simulink model "pid_control_V1"  (R2025b)
settings: Solver=FixedStepAuto  StartTime=0.0  StopTime=tsim  FixedStep=0.01  RelTol=1e-3
values from neighbouring files (symbols this model uses):
  Cp = 0.57    [Model.m]    (also in main_V1.m = 0.248)
  h_sp = 1.0    (= 1)    [main_V1.m]
  Kd_h = 5e-5    (= 5e-05)    [main_V1.m]
  Kd_pitch = 0.5    [main_V1.m]
  Ki_h = 1e-6    (= 1e-06)    [main_V1.m]
  Ki_pitch = 0.005    [main_V1.m]
  Kp_h = 1e-5    (= 1e-05)    [main_V1.m]
  Kp_pitch = 1.0    (= 1)    [main_V1.m]
  theta_sp = 2.5 * (pi/180)    (= 0.0436332312999)    [main_V1.m]
  Tp = 0.125*10^(-3)    (= 0.000125)    [Model.m]    (also in main_V1.m)
  u_nom = zeros(5,1)    [main_V1.m]
  x0 = x_nom    [main_V1.m]
undefined symbols (not defined in the file or in its folder): F, Light, MIL, state
libraries: aerolibactuator x5, ros2lib x2, slpidlib x2, robotcorelib x1, aerolibwind2 x1
settings Model: Creator=sofij  LastModifiedBy=facyu
settings SolverCC: AlgebraicLoopSolver=TrustRegion
settings OptimizationCC: DefaultParameterBehavior=Inlined  EnhancedBackFolding=on  PassReuseOutputArgsAs=Individual arguments  ZeroExternalMemoryAtStartup=off  ZeroInternalMemoryAtStartup=off  MaxStackSize=64  OptimizeBlockOrder=speed  DifferentSizesBufferReuse=on  OptimizationCustomize=off  EfficientTunableParamExpr=on
settings DebuggingCC: ParameterTunabilityLossMsg=error  UnconnectedInputMsg=warning  UnconnectedOutputMsg=warning  UnconnectedLineMsg=warning  SFUnexpectedBacktrackingDiag=warning  SFNoUnconditionalDefaultTransitionDiag=warning
settings HardwareCC: ProdBitPerLong=64.0  ProdHWDeviceType=Intel->x86-64 (Linux 64)  UseEmbeddedCoderFeatures=off
settings ModelReferenceCC: EnableRefExpFcnMdlSchedulingChecks=on
settings SFSimCC: MATLABDynamicMemAlloc=off
settings RTWCC: SystemTargetFile=ert.tlc  HardwareBoard=Robot Operating System 2 (ROS 2)  TLCOptions="-aInlineSetEventsForThisBaseRateFcn=TLC_FALSE -aSuppressMultiTaskScheduler=TLC_FALSE  -aRateBasedStepFcn=0"  TemplateMakefile=ert_default_tmf  GenerateReport=on  Toolchain=Colcon Tools  BuildConfiguration=Debug  LaunchReport=on  TargetLang=C++  GPUComputeCapability=3.5  DLArmComputeVersion=19.05  Description=Embedded Coder
settings CodeAppCC: ForceParamTrailComments=on  IgnoreCustomStorageClasses=off  OperatorAnnotations=on  SimulinkDataObjDesc=on  SFDataObjDesc=on  InsertBlockDesc=on  EnableCustomComments=on
settings ERTTargetCC: ExtModeTransport=2.0  ExtModeStaticAlloc=on  ExtModeAutomaticAllocSize=off  ExtModeMexFile=ext_xcp  ExtModeIntrfLevel=Level2 - Open  RootIOFormat=Structure reference  CodeInterfacePackaging=C++ class  SupportNonInlinedSFcns=on

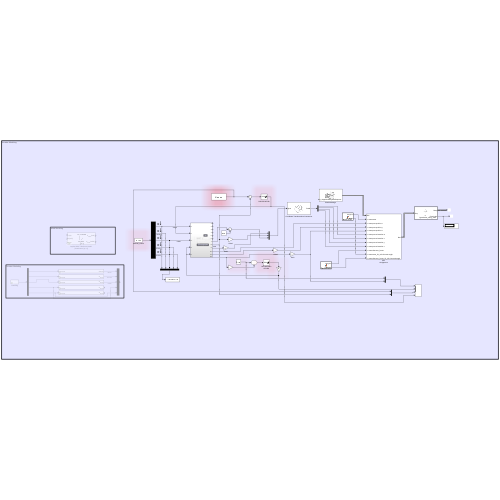
[thumbnail: Simulink's stored preview of the top-level diagram]
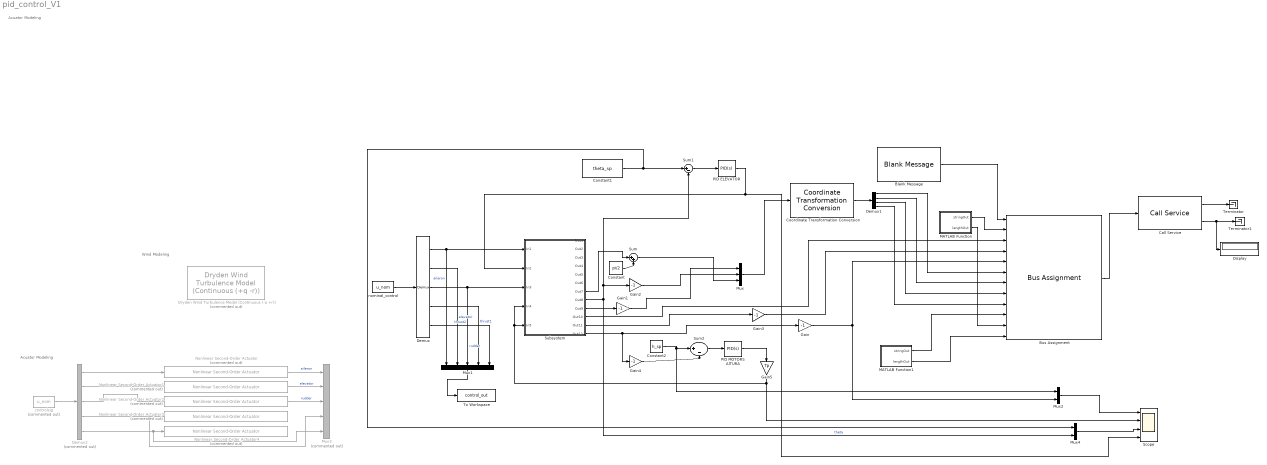
== system pid_control_V1 ==
  note: Wind Modeling
  note: Acuator Modeling
  note: Acuator Modeling
  Blank Message : ros2lib/Blank Message  messageClass=Service Request  entityType=gazebo_msgs/SetEntityState  messageType=gazebo_msgs/SetEntityStateRequest  SampleTime=0.01
  Bus Assignment : BusAssignment  AssignedSignals=state.name,state.pose.position.x,state.pose.position.y,state.pose.position.z,state.pose.orientation.w,state.pose.orientation.z,state.pose.orientation.y,state.pose.orientation.x,state.reference_frame,state.name_SL_Info.CurrentLength,state.reference_frame_SL_Info.CurrentLength
  Call Service : ros2lib/Call Service  topicSource=Specify your own  service=/gazebo/set_entity_state  serviceType=gazebo_msgs/SetEntityState  connectionTimeout=5  ShowErrorCodeOutput=on  legacyBusStruct=off  QOSHistory=Keep last  QOSDepth=1  QOSReliability=Reliable  QOSDurability=Volatile  QOSDeadline=Inf  QOSLifespan=Inf  QOSLiveliness=Automatic  QOSLeaseDuration=Inf  QOSAvoidROSNamespaceConventions=off
  Constant : Constant  Value=pi/2
  Constant1 : Constant  Value=theta_sp
  Constant2 : Constant  Value=h_sp
  Coordinate Transformation Conversion : robotcorelib/Coordinate Transformation Conversion  InputRepresentation=Euler Angles  InputEulerSequence=ZYX  ShowTrVecInputPort=on  OutputRepresentation=Quaternion  OutputEulerSequence=ZYX  ShowTrVecOutputPort=on  SimulateUsing=Interpreted execution
      settings: LibrarySourceBlock=roslib/Utilities/Coordinate Transformation Conversion
  Demux : Demux  Outputs=5
  Demux1 : Demux
  Demux2 : Demux  Commented=on  Outputs=5
  Display : Display
  Dryden Wind Turbulence Model (Continuous (-q +r)) : aerolibwind2/Dryden Wind Turbulence Model  (Continuous (+q -r))  Commented=on  units=Metric (MKS)  spec=MIL-F-8785C  model=Continuous Dryden (-q +r)  W20=15  Wdeg=0  TurbProb=10^-2 - Light  L_high=533.4  Wingspan=10  ts=0.1  Seed=[23341 23342 23343 23344]  T_on=on
  Gain{,1..4} (5 alike) : Gain  Gain=-1
  Gain5 : Gain  Gain=Tp
  MATLAB Function : MATLAB Function  TreatAsAtomicUnit=on
  MATLAB Function1 : MATLAB Function  TreatAsAtomicUnit=on
  Mux : Mux  Inputs=3
  Mux1 : Mux  Inputs=5
  Mux2 : Mux  Inputs=2
  Mux3 : Mux  Commented=on  Inputs=5
  Mux4 : Mux  Inputs=2
  Nonlinear Second-Order Actuator : aerolibactuator/Nonlinear Second-Order Actuator  Commented=on  wn_fin=1  z_fin=0.3  fin_max=15*pi/180  fin_min=-20*pi/180  fin_maxrate=500*pi/180  fin_act_0=0  fin_act_vel=0
  Nonlinear Second-Order Actuator1 : aerolibactuator/Nonlinear Second-Order Actuator  Commented=on  wn_fin=1  z_fin=0.3  fin_max=20*pi/180  fin_min=-20*pi/180  fin_maxrate=500*pi/180  fin_act_0=0  fin_act_vel=0
  Nonlinear Second-Order Actuator2 : aerolibactuator/Nonlinear Second-Order Actuator  Commented=on  wn_fin=1  z_fin=0.3  fin_max=15*pi/180  fin_min=-15*pi/180  fin_maxrate=500*pi/180  fin_act_0=0  fin_act_vel=0
  Nonlinear Second-Order Actuator3 : aerolibactuator/Nonlinear Second-Order Actuator  Commented=on  wn_fin=1  z_fin=0.3  fin_max=100  fin_min=0  fin_maxrate=500*pi/180  fin_act_0=0  fin_act_vel=0
  Nonlinear Second-Order Actuator4 : aerolibactuator/Nonlinear Second-Order Actuator  Commented=on  wn_fin=1  z_fin=0.3  fin_max=100  fin_min=0  fin_maxrate=500*pi/180  fin_act_0=0  fin_act_vel=0
  PID ELEVATOR : slpidlib/PID Controller  Controller=PID  Form=Parallel  TimeDomain=Continuous-time  UseExternalTs=off  SampleTime=-1  IntegratorMethod=Forward Euler  FilterMethod=Forward Euler  ControllerParametersSource=internal  P=Kp_pitch  I=Ki_pitch  UseKiTs=off  D=Kd_pitch  UseExternalDerivativeSource=off  N=100  UseFilter=on  TunerSelectOption=Transfer Function Based (PID Tuner App)  InitialConditionSource=internal  InitialConditionForIntegrator=0  InitialConditionForFilter=0  DifferentiatorICPrevScaledInput=0  ExternalReset=none  TrackingMode=off  Kt=1  LimitOutput=on  SatLimitsSource=internal  UpperSaturationLimit=20*pi/180  LowerSaturationLimit=-20*pi/180  LinearizeAsGain=on  AntiWindupMode=clamping  Kb=1  LimitIntegrator=off  UpperIntegratorSaturationLimit=inf  LowerIntegratorSaturationLimit=-inf  POutMin=[]  POutMax=[]  IOutMin=[]  IOutMax=[]  DOutMin=[]  DOutMax=[]  NOutMin=[]  NOutMax=[]  SumOutMin=[]  SumOutMax=[]  SaturationOutMin=[]  SaturationOutMax=[]  PParamMin=[]  PParamMax=[]  IParamMin=[]  IParamMax=[]  DParamMin=[]  DParamMax=[]  NParamMin=[]  NParamMax=[]  KbParamMin=[]  KbParamMax=[]  KtParamMin=[]  KtParamMax=[]  KbOutMin=[]  KbOutMax=[]  KtOutMin=[]  KtOutMax=[]  IntegratorOutMin=[]  IntegratorOutMax=[]  FilterOutMin=[]  FilterOutMax=[]  SumI1OutMin=[]  SumI1OutMax=[]  SumI2OutMin=[]  SumI2OutMax=[]  SumI3OutMin=[]  SumI3OutMax=[]  SumI4OutMin=[]  SumI4OutMax=[]  SumDOutMin=[]  SumDOutMax=[]  DifferentiatorOutMin=[]  DifferentiatorOutMax=[]  FilterDiffOutCoefMin=[]  FilterDiffOutCoefMax=[]  ReciprocalOutMin=[]  ReciprocalOutMax=[]  SumDenOutMin=[]  SumDenOutMax=[]  SumNumOutMin=[]  SumNumOutMax=[]  DivideOutMin=[]  DivideOutMax=[]  UdiffTsProdOutMin=[]  UdiffTsProdOutMax=[]  NTsProdOutMin=[]  NTsProdOutMax=[]  UintegralTsProdOutMin=[]  UintegralTsProdOutMax=[]  UngainTsProdOutMin=[]  UngainTsProdOutMax=[]  ClampingZeroOutDataTypeStr=Inherit: Inherit via back propagation  ClampingZeroOutMin=[]  ClampingZeroOutMax=[]  FilterDenConstantOutDataTypeStr=Inherit: Inherit via back propagation  FilterDenConstantOutMin=[]  FilterDenConstantOutMax=[]  PCopyOutDataTypeStr=Inherit: Inherit via back propagation  PCopyOutMin=[]  PCopyOutMax=[]  NCopyOutDataTypeStr=Inherit: Inherit via back propagation  NCopyOutMin=[]  NCopyOutMax=[]  IntegratorContinuousStateAttributes=''  IntegratorStateMustResolveToSignalObject=off  IntegratorRTWStateStorageClass=Auto  FilterContinuousStateAttributes=''  FilterStateMustResolveToSignalObject=off  FilterRTWStateStorageClass=Auto  ParallelPVariant=InternalParameters  IdealPVariant=Disabled  IVariant=InternalParameters  DVariant=InternalParameters  IntegratorVariant=Continuous  SatVariant=Enabled  AWVariant=ContClampingParallel  PCopyVariant=Disabled  TRVariant=Disabled  FdbkBlocksVariant=Forward  IdealPFdbkVariant=Disabled  SatFdbkVariant=Disabled  DerivativeFilterVariant=ContFilter  NVariant=InternalParameters  NCopyVariant=Disabled  FilterICVariant=InternalICsFilter  IntegratorICVariant=InternalICs  ExternalResetVariant=Disabled  TRSumVariant=Passthrough  SumFdbkVariant=Disabled  SumVariant=Sum_PID  TsampFilterVariant=InternalTs  TsampNgainVariant=Passthrough  TsampIntegralVariant=Disabled_SignalSpec  ExternalSaturationOutDataTypeStr=Inherit: Same as second input  DerivativeSourceVariant=ErrorSignal  PreIntVariant=InternalPreInt
  PID MOTORS AlTURA : slpidlib/PID Controller  Controller=PID  Form=Parallel  TimeDomain=Continuous-time  UseExternalTs=off  SampleTime=-1  IntegratorMethod=Forward Euler  FilterMethod=Forward Euler  ControllerParametersSource=internal  P=Kp_h  I=Ki_h  UseKiTs=off  D=Kd_h  UseExternalDerivativeSource=off  N=100  UseFilter=on  TunerSelectOption=Transfer Function Based (PID Tuner App)  InitialConditionSource=internal  InitialConditionForIntegrator=0  InitialConditionForFilter=0  DifferentiatorICPrevScaledInput=0  ExternalReset=none  TrackingMode=off  Kt=1  LimitOutput=on  SatLimitsSource=internal  UpperSaturationLimit=1  LowerSaturationLimit=0  LinearizeAsGain=on  AntiWindupMode=clamping  Kb=1  LimitIntegrator=off  UpperIntegratorSaturationLimit=inf  LowerIntegratorSaturationLimit=-inf  POutMin=[]  POutMax=[]  IOutMin=[]  IOutMax=[]  DOutMin=[]  DOutMax=[]  NOutMin=[]  NOutMax=[]  SumOutMin=[]  SumOutMax=[]  SaturationOutMin=[]  SaturationOutMax=[]  PParamMin=[]  PParamMax=[]  IParamMin=[]  IParamMax=[]  DParamMin=[]  DParamMax=[]  NParamMin=[]  NParamMax=[]  KbParamMin=[]  KbParamMax=[]  KtParamMin=[]  KtParamMax=[]  KbOutMin=[]  KbOutMax=[]  KtOutMin=[]  KtOutMax=[]  IntegratorOutMin=[]  IntegratorOutMax=[]  FilterOutMin=[]  FilterOutMax=[]  SumI1OutMin=[]  SumI1OutMax=[]  SumI2OutMin=[]  SumI2OutMax=[]  SumI3OutMin=[]  SumI3OutMax=[]  SumI4OutMin=[]  SumI4OutMax=[]  SumDOutMin=[]  SumDOutMax=[]  DifferentiatorOutMin=[]  DifferentiatorOutMax=[]  FilterDiffOutCoefMin=[]  FilterDiffOutCoefMax=[]  ReciprocalOutMin=[]  ReciprocalOutMax=[]  SumDenOutMin=[]  SumDenOutMax=[]  SumNumOutMin=[]  SumNumOutMax=[]  DivideOutMin=[]  DivideOutMax=[]  UdiffTsProdOutMin=[]  UdiffTsProdOutMax=[]  NTsProdOutMin=[]  NTsProdOutMax=[]  UintegralTsProdOutMin=[]  UintegralTsProdOutMax=[]  UngainTsProdOutMin=[]  UngainTsProdOutMax=[]  ClampingZeroOutDataTypeStr=Inherit: Inherit via back propagation  ClampingZeroOutMin=[]  ClampingZeroOutMax=[]  FilterDenConstantOutDataTypeStr=Inherit: Inherit via back propagation  FilterDenConstantOutMin=[]  FilterDenConstantOutMax=[]  PCopyOutDataTypeStr=Inherit: Inherit via back propagation  PCopyOutMin=[]  PCopyOutMax=[]  NCopyOutDataTypeStr=Inherit: Inherit via back propagation  NCopyOutMin=[]  NCopyOutMax=[]  IntegratorContinuousStateAttributes=''  IntegratorStateMustResolveToSignalObject=off  IntegratorRTWStateStorageClass=Auto  FilterContinuousStateAttributes=''  FilterStateMustResolveToSignalObject=off  FilterRTWStateStorageClass=Auto  ParallelPVariant=InternalParameters  IdealPVariant=Disabled  IVariant=InternalParameters  DVariant=InternalParameters  IntegratorVariant=Continuous  SatVariant=Enabled  AWVariant=ContClampingParallel  PCopyVariant=Disabled  TRVariant=Disabled  FdbkBlocksVariant=Forward  IdealPFdbkVariant=Disabled  SatFdbkVariant=Disabled  DerivativeFilterVariant=ContFilter  NVariant=InternalParameters  NCopyVariant=Disabled  FilterICVariant=InternalICsFilter  IntegratorICVariant=InternalICs  ExternalResetVariant=Disabled  TRSumVariant=Passthrough  SumFdbkVariant=Disabled  SumVariant=Sum_PID  TsampFilterVariant=InternalTs  TsampNgainVariant=Passthrough  TsampIntegralVariant=Disabled_SignalSpec  ExternalSaturationOutDataTypeStr=Inherit: Same as second input  DerivativeSourceVariant=ErrorSignal  PreIntVariant=InternalPreInt
  Scope : Scope  NumInputPorts=4
      settings: ActiveDisplayYMinimum=-78.933080548030773  ActiveDisplayYMaximum=231.90042697188215  DataLoggingVariableName=ScopeData4
  Subsystem : Subsystem
  Sum : Sum  Inputs=|++
  Sum1 : Sum  Inputs=|+-
  Sum2 : Sum  Inputs=|+-
  Terminator : Terminator
  Terminator1 : Terminator
  To Workspace : ToWorkspace  VariableName=control_out  SampleTime=-1
      settings: Save2DSignal=2-D array (concatenate along first dimension)
  controlsig : Constant  Commented=on  Value=u_nom
  nominal_control : Constant  Value=u_nom
  wires:
  controlsig/1 -> Demux2/1
  Nonlinear Second-Order Actuator/1 -> Mux3/1  "aileron"
  Demux2/1 -> Nonlinear Second-Order Actuator/1
  Demux2/5 -> Mux3/5, Nonlinear Second-Order Actuator4/1
  Demux2/4 -> Mux3/4, Nonlinear Second-Order Actuator3/1
  Demux2/3 -> Nonlinear Second-Order Actuator2/1
  Demux2/2 -> Nonlinear Second-Order Actuator1/1
  Nonlinear Second-Order Actuator2/1 -> Mux3/3  "rudder"
  Nonlinear Second-Order Actuator1/1 -> Mux3/2  "elevator"
  Demux/3 -> Mux1/3, Subsystem/3(In3)  "rudder"
  nominal_control/1 -> Demux/1
  Demux/1 -> Subsystem/1(In1), Mux1/1  "aileron"
  Blank Message/1 -> Bus Assignment/1
  Subsystem/10(Out10) -> Bus Assignment/3
  Subsystem/11(Out11) -> Gain3/1
  Subsystem/12(Out12) -> Gain4/1, Gain/1
  Subsystem/8(Out8) -> Mux4/2, Gain2/1, Sum1/2  "theta"
  Subsystem/9(Out9) -> Gain1/1
  Mux/1 -> Coordinate Transformation Conversion/1
  Coordinate Transformation Conversion/1 -> Demux1/1
  Demux1/1 -> Bus Assignment/6
  Demux1/2 -> Bus Assignment/7
  Demux1/3 -> Bus Assignment/8
  Demux1/4 -> Bus Assignment/9
  Bus Assignment/1 -> Call Service/1
  Gain/1 -> Mux2/2, Bus Assignment/5
  Call Service/1 -> Terminator/1
  Call Service/2 -> Display/1, Terminator1/1
  MATLAB Function/1(stringOut) -> Bus Assignment/2
  MATLAB Function1/1(stringOut) -> Bus Assignment/10
  MATLAB Function/2(lengthOut) -> Bus Assignment/11
  MATLAB Function1/2(lengthOut) -> Bus Assignment/12
  Gain2/1 -> Mux/2
  Subsystem/7(Out7) -> Sum/1
  Gain3/1 -> Bus Assignment/4
  Gain1/1 -> Mux/1
  Sum/1 -> Mux/3
  Constant/1 -> Sum/2
  Constant1/1 -> Sum1/1, Mux4/1
  Sum1/1 -> PID ELEVATOR/1
  PID ELEVATOR/1 -> Scope/4, Subsystem/2(In2)
  Constant2/1 -> Mux2/1, Sum2/1
  Gain4/1 -> Sum2/2
  Sum2/1 -> PID MOTORS AlTURA/1
  PID MOTORS AlTURA/1 -> Gain5/1
  Mux2/1 -> Scope/1
  Mux4/1 -> Scope/3
  Gain5/1 -> Subsystem/5(In5), Subsystem/4(In4), Scope/2
  Mux1/1 -> To Workspace/1
  Demux/2 -> Mux1/2  "elevator"
  Demux/4 -> Mux1/4  "thrust1"
  Demux/5 -> Mux1/5  "thrust2"

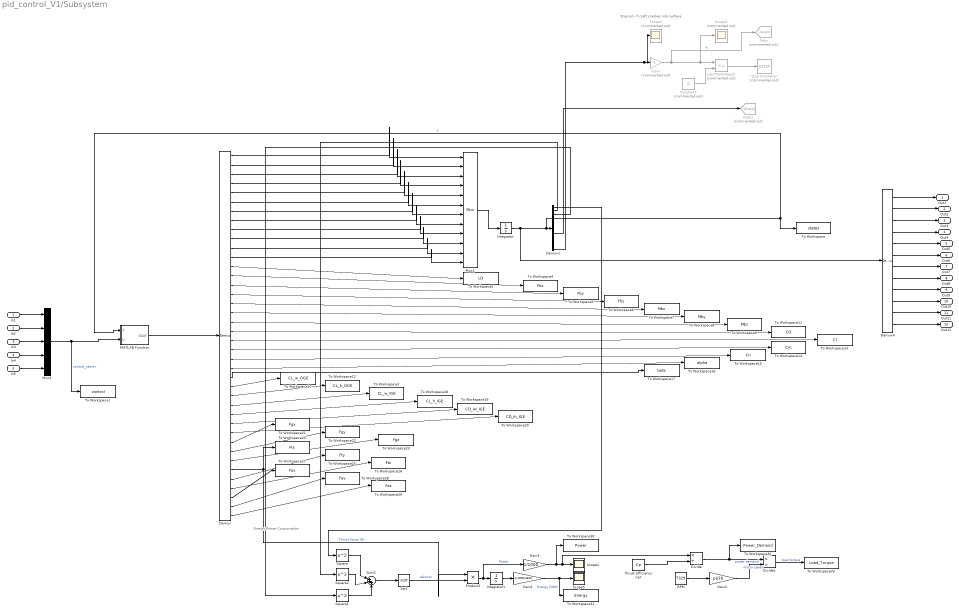
== system pid_control_V1/Subsystem ==
  note: Stop sim if craft crashes into surface
  note: Energy/Power Consumption
  In1 : Inport
  In2 : Inport  Port=2
  In3 : Inport  Port=3
  In4 : Inport  Port=4
  In5 : Inport  Port=5
  Constant1 : Constant  Commented=on  Value=0
  Demux : Demux  Outputs=40
  Demux1 : Demux  Outputs=12
  Demux4 : Demux  Outputs=12
  Divide : Product  Inputs=*/
  Divide1 : Product  Inputs=*/
  Gain : Gain  Commented=on  Gain=-1
  Gain1 : Gain  Gain=1/1000/3600
  Gain2 : Gain  Gain=pi/30
  Gain3 : Gain  Gain=1/1000
  Goto : Goto  Commented=on  GotoTag=height
  Goto1 : Goto  Commented=on  GotoTag=theta
  Integrator : Integrator  InitialCondition=x0
  Integrator1 : Integrator
  LessThanOrEqual : RelationalOperator  Commented=on  Operator=<=  OutDataTypeStr=boolean  RndMeth=Simplest  InputSameDT=off
  MATLAB Function : MATLAB Function  TreatAsAtomicUnit=on
  Mux1 : Mux  Inputs=12
  Mux4 : Mux  Inputs=5
  Product2 : Product
  RPM : Constant  Value=7329
  Scope2 : Scope  Commented=on
      settings: ActiveDisplayYMinimum=-1.36989  ActiveDisplayYMaximum=0.16067
  Scope3 : Scope  Commented=on
      settings: ActiveDisplayYMinimum=-0.16067  ActiveDisplayYMaximum=1.36989  DataLoggingVariableName=ScopeData2
  Scope4 : Scope
      settings: ActiveDisplayYMinimum=-1  ActiveDisplayYMaximum=1  DataLoggingVariableName=ScopeData3
  Scope5 : Scope
  Sqrt : Sqrt
  Square : Math  Operator=square
  Square1 : Math  Operator=square
  Square2 : Math  Operator=square
  Stop Simulation : Stop  Commented=on
  Sum2 : Sum  Inputs=|+++
  To Workspace : ToWorkspace  VariableName=states  SampleTime=-1
  To Workspace1 : ToWorkspace  VariableName=control  SampleTime=-1
  To Workspace10 : ToWorkspace  VariableName=CL_w_OGE  SampleTime=-1
      settings: Save2DSignal=2-D array (concatenate along first dimension)
  To Workspace11 : ToWorkspace  VariableName=CQ  SampleTime=-1
      settings: Save2DSignal=2-D array (concatenate along first dimension)
  To Workspace12 : ToWorkspace  VariableName=CL_h_OGE  SampleTime=-1
      settings: Save2DSignal=2-D array (concatenate along first dimension)
  To Workspace13 : ToWorkspace  VariableName=Cl  SampleTime=-1
      settings: Save2DSignal=2-D array (concatenate along first dimension)
  To Workspace14 : ToWorkspace  VariableName=Cm  SampleTime=-1
      settings: Save2DSignal=2-D array (concatenate along first dimension)
  To Workspace15 : ToWorkspace  VariableName=Cn  SampleTime=-1
      settings: Save2DSignal=2-D array (concatenate along first dimension)
  To Workspace16 : ToWorkspace  VariableName=alpha  SampleTime=-1
      settings: Save2DSignal=2-D array (concatenate along first dimension)
  To Workspace17 : ToWorkspace  VariableName=beta  SampleTime=-1
      settings: Save2DSignal=2-D array (concatenate along first dimension)
  To Workspace18 : ToWorkspace  VariableName=CL_h_IGE  SampleTime=-1
      settings: Save2DSignal=2-D array (concatenate along first dimension)
  To Workspace19 : ToWorkspace  VariableName=CD_iw_IGE  SampleTime=-1
      settings: Save2DSignal=2-D array (concatenate along first dimension)
  To Workspace2 : ToWorkspace  VariableName=LD  SampleTime=-1
      settings: Save2DSignal=2-D array (concatenate along first dimension)
  To Workspace20 : ToWorkspace  VariableName=CD_ih_IGE  SampleTime=-1
      settings: Save2DSignal=2-D array (concatenate along first dimension)
  To Workspace21 : ToWorkspace  VariableName=Fgx  SampleTime=-1
      settings: Save2DSignal=2-D array (concatenate along first dimension)
  To Workspace22 : ToWorkspace  VariableName=Fgy  SampleTime=-1
      settings: Save2DSignal=2-D array (concatenate along first dimension)
  To Workspace23 : ToWorkspace  VariableName=Fgz  SampleTime=-1
      settings: Save2DSignal=2-D array (concatenate along first dimension)
  To Workspace24 : ToWorkspace  VariableName=Ftx  SampleTime=-1
      settings: Save2DSignal=2-D array (concatenate along first dimension)
  To Workspace25 : ToWorkspace  VariableName=Fty  SampleTime=-1
      settings: Save2DSignal=2-D array (concatenate along first dimension)
  To Workspace26 : ToWorkspace  VariableName=Ftz  SampleTime=-1
      settings: Save2DSignal=2-D array (concatenate along first dimension)
  To Workspace27 : ToWorkspace  VariableName=Fax  SampleTime=-1
      settings: Save2DSignal=2-D array (concatenate along first dimension)
  To Workspace28 : ToWorkspace  VariableName=Fay  SampleTime=-1
      settings: Save2DSignal=2-D array (concatenate along first dimension)
  To Workspace29 : ToWorkspace  VariableName=Faz  SampleTime=-1
      settings: Save2DSignal=2-D array (concatenate along first dimension)
  To Workspace3 : ToWorkspace  VariableName=CL_w_IGE  SampleTime=-1
      settings: Save2DSignal=2-D array (concatenate along first dimension)
  To Workspace30 : ToWorkspace  VariableName=Power  SampleTime=-1
      settings: Save2DSignal=2-D array (concatenate along first dimension)
  To Workspace31 : ToWorkspace  VariableName=Energy  SampleTime=-1
      settings: Save2DSignal=2-D array (concatenate along first dimension)
  To Workspace32 : ToWorkspace  VariableName=Power_Demand  SampleTime=-1
      settings: Save2DSignal=2-D array (concatenate along first dimension)
  To Workspace33 : ToWorkspace  VariableName=Load_Torque  SampleTime=-1
      settings: Save2DSignal=2-D array (concatenate along first dimension)
  To Workspace4 : ToWorkspace  VariableName=Fbx  SampleTime=-1
      settings: Save2DSignal=2-D array (concatenate along first dimension)
  To Workspace5 : ToWorkspace  VariableName=Fby  SampleTime=-1
      settings: Save2DSignal=2-D array (concatenate along first dimension)
  To Workspace6 : ToWorkspace  VariableName=Fbz  SampleTime=-1
      settings: Save2DSignal=2-D array (concatenate along first dimension)
  To Workspace7 : ToWorkspace  VariableName=Mbx  SampleTime=-1
      settings: Save2DSignal=2-D array (concatenate along first dimension)
  To Workspace8 : ToWorkspace  VariableName=Mby  SampleTime=-1
      settings: Save2DSignal=2-D array (concatenate along first dimension)
  To Workspace9 : ToWorkspace  VariableName=Mbz  SampleTime=-1
      settings: Save2DSignal=2-D array (concatenate along first dimension)
  thrust efficiency Cp? : Constant  Value=Cp
  Out1 : Outport
  Out2 : Outport  Port=2
  Out3 : Outport  Port=3
  Out4 : Outport  Port=4
  Out5 : Outport  Port=5
  Out6 : Outport  Port=6
  Out7 : Outport  Port=7
  Out8 : Outport  Port=8
  Out9 : Outport  Port=9
  Out10 : Outport  Port=10
  Out11 : Outport  Port=11
  Out12 : Outport  Port=12
  wires:
  Demux4/3 -> Out3/1
  Mux4/1 -> MATLAB Function/2(U), To Workspace1/1  "control_vector"
  In1/1 -> Mux4/1
  Product2/1 -> Gain3/1, Integrator1/1  "Power"
  Demux/27 -> To Workspace12/1
  Demux/31 -> To Workspace20/1
  Demux/4 -> Mux1/4
  Demux/33 -> To Workspace22/1
  Demux1/8 -> Goto1/1
  Divide/1 -> To Workspace32/1, Divide1/1  "power demand"
  Gain1/1 -> To Workspace31/1, Scope5/1  "Energy (kWh)"
  Demux1/2 -> Square2/1
  Demux/8 -> Mux1/8
  LessThanOrEqual/1 -> Stop Simulation/1
  RPM/1 -> Gain2/1
  Demux/2 -> Mux1/2
  Demux/21 -> To Workspace13/1
  Demux/29 -> To Workspace18/1
  Demux/22 -> To Workspace14/1
  Demux/36 -> To Workspace25/1
  Demux/38 -> To Workspace27/1
  Demux/40 -> To Workspace29/1
  Demux/28 -> To Workspace3/1
  Demux/17 -> To Workspace7/1
  Gain3/1 -> To Workspace30/1, Divide/1, Scope4/1
  Demux1/3 -> Square1/1
  Demux/18 -> To Workspace8/1
  Divide1/1 -> To Workspace33/1  "load torque"
  Constant1/1 -> LessThanOrEqual/2
  Sqrt/1 -> Product2/2  "velocity"
  Square2/1 -> Sum2/2
  Square1/1 -> Sum2/3
  Demux/39 -> To Workspace28/1
  Gain2/1 -> Divide1/2  "motor speed"
  Demux/25 -> To Workspace17/1
  Demux/23 -> To Workspace15/1
  Demux/9 -> Mux1/9
  Demux1/1 -> Square/1
  Demux/26 -> To Workspace10/1
  Square/1 -> Sum2/1
  thrust efficiency Cp?/1 -> Divide/2
  Demux/14 -> To Workspace4/1
  Demux/15 -> To Workspace5/1
  Sum2/1 -> Sqrt/1
  Demux/11 -> Mux1/11
  Demux/37 -> To Workspace26/1
  Demux/19 -> To Workspace9/1
  Gain/1 -> Goto/1, Scope3/1, LessThanOrEqual/1  "h"
  Demux/20 -> To Workspace11/1
  Demux/7 -> Mux1/7
  Demux/3 -> Mux1/3
  MATLAB Function/1(XDOT) -> Demux/1
  Demux/35 -> Product2/1, To Workspace24/1  "Thrust Force (N)"
  Integrator/1 -> Demux4/1, To Workspace/1, MATLAB Function/1(X), Demux1/1  "x"
  Demux/24 -> To Workspace16/1
  Demux/6 -> Mux1/6
  Demux/5 -> Mux1/5
  Mux1/1 -> Integrator/1
  Demux/30 -> To Workspace19/1
  In5/1 -> Mux4/5
  In4/1 -> Mux4/4
  Demux/1 -> Mux1/1
  In2/1 -> Mux4/2
  Demux/10 -> Mux1/10
  Demux4/11 -> Out11/1
  Demux4/6 -> Out6/1
  Demux/13 -> To Workspace2/1
  Demux4/2 -> Out2/1
  Demux4/9 -> Out9/1
  Demux4/1 -> Out1/1
  Integrator1/1 -> Gain1/1
  Demux4/4 -> Out4/1
  Demux/34 -> To Workspace23/1
  Demux4/10 -> Out10/1
  Demux4/8 -> Out8/1
  Demux/12 -> Mux1/12
  Demux/16 -> To Workspace6/1
  Demux/32 -> To Workspace21/1
  Demux4/5 -> Out5/1
  Demux1/12 -> Scope2/1, Gain/1
  In3/1 -> Mux4/3
  Demux4/7 -> Out7/1
  Demux4/12 -> Out12/1

== matlab function pid_control_V1/Subsystem/MATLAB Function ==
  data: X input; XDOT output; U input
function XDOT  = Model(X,U)
%#codegen

%-----------STATE AND CONTROL VECTORS-------------
x1 = X(1); %u
x2 = X(2); %v
x3 = X(3); %w
x4 = X(4); %p
x5 = X(5); %q
x6 = X(6); %r
x7 = X(7); %phi
x8 = X(8); %theta
x9 = X(9); %psi
x10 = X(10); % x_NED
x11 = X(11); % y_NED
x12 = X(12); % z_NED

u1 = U(1); %d_A (Aileron)
u2 = U(2); %d_E (Elevator)
u3 = U(3); %d_R (Rudder)
u4 = U(4); %d_th1 (throttle 1)
u5 = U(5); %d_th2 (throttle 2)

%-----------SYSTEM PARAMETERS------------------------------
m = 112; % Aircraft mass (Kg)
vc = 28; % cruise speed
bw = 5.02; % Span (Wing)
bh = 2.74; % Span (HTP)
cbar = 0.646; % Mean Aerodynamic Chord (m)
lt = 24.8;  % Distance of AC of tail and body (m)
Sw = 3.334;    % Wing planform area (m^2)
Sh = 1.128;    % Tail planform area (m^2)
ARw = 7.5; % Apect Ratio (Wing) 
ARh = 6.7; % Apect Ratio (HTP) 
TRw = 0.4; % Taper Ratio (Wing) 
TRh = 0.5; % Taper Ratio (HTP) 

Xcg = 0;  % x position of CG in Fm (m)
Ycg = 0;  % y position of CG in Fm (m)
Zcg = 0;  % z position of CG in Fm (m)

Xac = 0.097;  % x position of Aerodynamic Center in Fm (m)
Yac = 0;      % y position of Aerodynamic Center in Fm (m)
Zac = -0.06;  % z position of Aerodynamic Center in Fm (m)

%Engine constants

Xapt1 = -0.519; % x position of engine 1 force in Fm (m)
Yapt1 = 0.6;    % y position of engine 1 force in Fm (m)
Zapt1 = 0.285;  % z position of engine 1 force in Fm (m)

Xapt2 = -0.519;  % x position of engine 2 force in Fm (m)
Yapt2 = -0.6;    % y position of engine 2 force in Fm (m)
Zapt2 = 0.285;   % z position of engine 2 force in Fm (m)

%Other constants
rho = 1.225;
g = 9.81;
e0w = 0.9; % Oswald's efficiency Factor (Wing)
e0h = 0.9; % Oswald's efficiency Factor (HTP)
alpha_0w = -3.75*pi/180; % Zero Lift Angle of Attack (Wing)
alpha_0h = -4.25*pi/180; % Zero Lift Angle of Attack (HTP)
iw = 4.75*pi/180; % Angle of incidence (Wing)
ih = 2.5*pi/180; % Angle of Incidence (HTP)
eps = 0; % Downwash Angle
zw = 0.363; % Wing Offset
zh = 0.72; % HTP Offset
CD_0 = 0.0306; % Zero Lift Drag Coefficient
Tp = 0.125*10^(-3); % motor PWM switching frequency

%-----------CONTROL LIMITS SATURATION------------------------------

% aileron
u1min = -20*pi/180;
u1max =  15*pi/180;

% elevator
u2min = -20*pi/180;
u2max =  20*pi/180;

% rudder
u3min = -15*pi/180;
u3max =  15*pi/180;

% engines 
u4min =  0;
u4max =  Tp;

u5min =  0;
u5max = Tp;

if(u1>u1max)
    u1=u1max;
elseif(u1<u1min)
    u1=u1min;
end

if(u2>u2max)
    u2=u2max;
elseif(u2<u2min)
    u2=u2min;
end

if(u3>u3max)
    u3=u3max;
elseif(u3<u3min)
    u3=u3min;
end

if(u4>u4max)
    u4=u4max;
elseif(u4<u4min)
    u4=u4min;
end

if(u5>u5max)
    u5=u5max;
elseif(u5<u5min)
    u5=u5min;
end

%-------------INTERMEDIATE VARIABLES-----------------------------

u = x1; 
v = x2; 
w = x3;
phi = x7; 
theta = x8; 
psi = x9;
c_phi = cos(phi);
s_phi = sin(phi);
c_theta = cos(theta);
s_theta = sin(theta);
c_psi = cos(psi);
s_psi = sin(psi);

% rotation matrix
Rb_v = [c_theta*c_psi c_theta*s_psi -s_theta;
        s_phi*s_theta*c_psi-c_phi*s_psi s_phi*s_theta*s_psi+c_phi*c_psi s_phi*c_theta;
        c_phi*s_theta*c_psi+s_phi*s_psi c_phi*s_theta*s_psi-s_phi*c_psi c_phi*c_theta];

Vb_g = [u;v;w];

% steady-state component of wind
w_ns = 0;
w_es = 0;
w_ds = 0;

% gust component of wind
u_wg = 0;
v_wg = 0;
w_wg = 0;

Vb_w = Rb_v*[w_ns;w_es;w_ds]+[u_wg;v_wg;w_wg];

Va_b = [Vb_g(1)-Vb_w(1);Vb_g(2)-Vb_w(2);Vb_g(3)-Vb_w(3)];

u_r = Va_b(1);
v_r = Va_b(2);
w_r = Va_b(3);

Va = sqrt(u_r^2+v_r^2+w_r^2);
alpha = atan2(w_r,u_r);
beta = asin(v_r/Va);

h = -x12;
hw = h-zw; % wing below CG -> h-offset
hh = h+zh; % tail above CG -> h+offset

Q = 0.5*rho*Va^2;     %dynamic pressure

wbe_b = [x4;x5;x6];
V_b = [x1;x2;x3];

%--------------Aerodynamic Force Coefficients---------------------

% Lift
mu_Lw = 1 + (1 - 2.25 * (TRw^0.00273 - 0.997)*((ARw^0.717)+13.6))*(288 * abs(hw/bw)^0.787 * exp(-9.14*(abs(hw/bw)^0.327)))/(ARw^0.882);
mu_Lh = 1 + (1 - 2.25 * (TRh^0.00273 - 0.997)*((ARh^0.717)+13.6))*(288 * abs(hh/bh)^0.787 * exp(-9.14*(abs(hh/bh)^0.327)))/(ARh^0.882);

C_L_e = -0.00141*u2^2+0.0307*u2;

CL_w_OGE = 2*pi*(ARw/(ARw+2))*(alpha-alpha_0w+iw);
CL_h_OGE = 2*pi*(ARh/(ARh+2))*(alpha-alpha_0h+ih+eps);

CL_w_IGE = CL_w_OGE*mu_Lw;
CL_h_IGE = (CL_h_OGE + C_L_e)*mu_Lh;

% Drag
mu_Dw = 1 - exp(-10.1*(abs(hw/bw)^0.686));
mu_Dh = 1 - exp(-10.1*(abs(hh/bh)^0.686));

CD_iw_OGE = (CL_w_OGE^2)/(pi*ARw*e0w);
CD_ih_OGE = (CL_h_OGE^2)/(pi*ARh*e0h);

CD_iw_IGE = CD_iw_OGE*mu_Dw;
CD_ih_IGE = CD_ih_OGE*mu_Dh;

CD_tot_wIGE = CD_0 + CD_iw_IGE;
CD_tot_hIGE = CD_0 + CD_ih_IGE;

LD_ratio = CL_w_IGE / CD_tot_wIGE;

% Total drag
CD_tot = CD_tot_wIGE + CD_tot_hIGE;
Dtot = CD_tot*Q*Sw;
Ltot = (CL_w_IGE*Sw + CL_h_IGE*Sh)*Q;

CQ = 0; % Assuming this wasn't implemented

FA_s = [-Dtot;
         CQ*Q*Sw;
        -Ltot];

C_bs = [cos(alpha) 0 -sin(alpha);0 1 0;sin(alpha) 0 cos(alpha)]; % rotation matrix
FA_b = C_bs*FA_s;

% steady-state
Cl = -0.0005*beta*180/pi;
Cm = -0.02*alpha*180/pi;
Cn = -0.002*beta*180/pi;
CMac_b = [Cl;Cm;Cn];

%-------------------------6. Aero moment about CG--------------------------
MAcg_b = CMac_b.*[bw*Q*Sw;cbar*Q*Sw;bw*Q*Sw];

%-------------------------8. Engine Force & Moment-------------------------
km = 37.42;
Cp = 0.57;
D = 0.635; 
Sp = pi*(D^2/4); 

d_t1 = u4/Tp; 
Vd1 = Va + d_t1*(km-Va);
Tp1 = 0.5*rho*Sp*Cp*Vd1*(Vd1-Va);

d_t2 = u5/Tp; 
Vd2 = Va + d_t2*(km-Va);
Tp2 = 0.5*rho*Sp*Cp*Vd2*(Vd2-Va);

FE1_b = [Tp1*cos(-5*pi/180);
         0;
         sin(5*pi/180)];
         
FE2_b = [Tp2*cos(-5*pi/180);
         0;
         sin(5*pi/180)];
         
FE_b = FE1_b + FE2_b;

mew1 = [Xcg-Xapt1;
        Yapt1-Ycg;
        Zcg-Zapt1];
        
mew2 = [Xcg-Xapt2;
        Yapt2-Ycg;
        Zcg-Zapt2];
        
MEcg1_b = cross(mew1,FE1_b);
MEcg2_b = cross(mew2,FE2_b);
MEcg_b = MEcg1_b + MEcg2_b;

%----------------------------9. Gravity Effect-----------------------------
g_b = [-g*sin(x8);g*cos(x8)*sin(x7);g*cos(x8)*cos(x7)];
Fg_b = m*g_b;

%----------------------------10. State Derivatives------------------------
% Inertia Matrix and its Inverse (Pre-calculated for C-Code generation)
% Ib = [39.71 0 8.97; 0 85.51 0; 8.97 0 114.39];
invIb = [0.0256247963 0 -0.0020093863;
         0            0.0116945386 0;
        -0.0020093863 0            0.0088954752]; 

F_b = Fg_b + FE_b + FA_b;
x1to3dot = (1/m)*F_b - cross(wbe_b,V_b);

Mcg_b = MAcg_b + MEcg_b;
% Using Ib directly for cross product
Ib_wbe_b = [39.71*x4 + 8.97*x6;
            85.51*x5;
            8.97*x4 + 114.39*x6];

x4to6dot = invIb*(Mcg_b - cross(wbe_b, Ib_wbe_b));

% MFS
H_phi = [1 0 0;
         0 cos(alpha) -sin(beta);
         0 sin(alpha) cos(alpha)];
         
x7to9dot = H_phi*wbe_b;
x10to12dot = rot_body_to_ned(X(1:9));

XDOT = [x1to3dot;
        x4to6dot;
        x7to9dot;
        x10to12dot;
        LD_ratio;
        F_b;
        Mcg_b;
        CQ;
        Cl;
        Cm;
        Cn;
        alpha;
        beta;
        CL_w_OGE;
        CL_h_OGE;
        CL_w_IGE;
        CL_h_IGE;
        CD_iw_IGE;
        CD_ih_IGE;
        Fg_b;
        FE_b; 
        FA_b];
end

%------------------------- LOCAL FUNCTIONS -------------------------
function [V_NED] = rot_body_to_ned(X)
%#codegen
V_body=[X(1);X(2);X(3)];

yaw=X(7); % phi
pitch=X(8); % theta
roll=X(9); % psi

R=[cos(pitch)*cos(yaw) cos(yaw)*sin(pitch)*sin(roll)-sin(yaw)*cos(roll) sin(roll)*sin(yaw)+sin(pitch)*cos(yaw)*cos(roll);
   cos(pitch)*sin(yaw) cos(yaw)*cos(roll)+sin(yaw)*sin(pitch)*sin(roll) sin(pitch)*sin(yaw)*cos(roll)-cos(yaw)*sin(roll);
  -sin(pitch)          sin(roll)*cos(pitch)                             cos(pitch)*cos(roll)];

V_NED=R'*V_body;
V_NED=[V_NED(1);V_NED(2);V_NED(3)];
end

== matlab function pid_control_V1/MATLAB Function1 ==
  data: stringOut output; lengthOut output
function [stringOut, lengthOut] = frameToROS()

    % Define el marco de referencia
    miTexto = 'world';
    
    % Crea el vector columna de 128 ceros tipo uint8
    stringOut = zeros(128, 1, 'uint8');
    
    % Copia las letras de 'world' al inicio
    stringOut(1:length(miTexto)) = uint8(miTexto);
    
    % Calcula la longitud exacta para ROS 2
    lengthOut = uint32(length(miTexto));

end

== matlab function pid_control_V1/MATLAB Function ==
  data: stringOut output; lengthOut output
function [stringOut, lengthOut] = stringToROS()
    
    % Define la palabra exacta (fíjate que sea el mismo nombre que en el .world)
    miTexto = 'ekranoplano';
    
    % Crea el vector de 128 posiciones
    stringOut = zeros(128, 1, 'uint8');
    stringOut(1:length(miTexto)) = uint8(miTexto);
    
    % Calcula la longitud para ROS (en tipo uint32)
    lengthOut = uint32(length(miTexto));
    
end
